simulink model "SimplePendulum"  (R2025b)
settings: Solver=VariableStepAuto  StartTime=0.0  StopTime=10.0  RelTol=1e-3
settings Model: Creator=alvaro  LastModifiedBy=alvaro

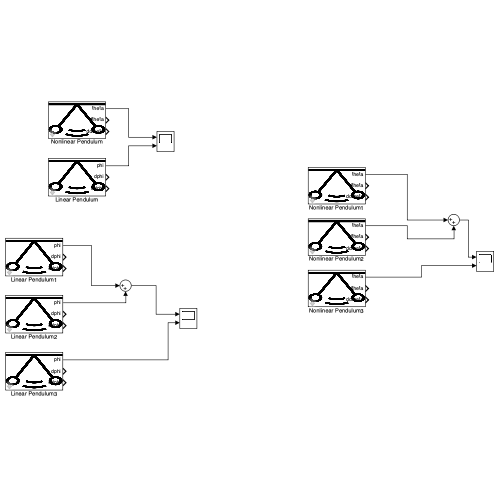
[thumbnail: Simulink's stored preview of the top-level diagram]
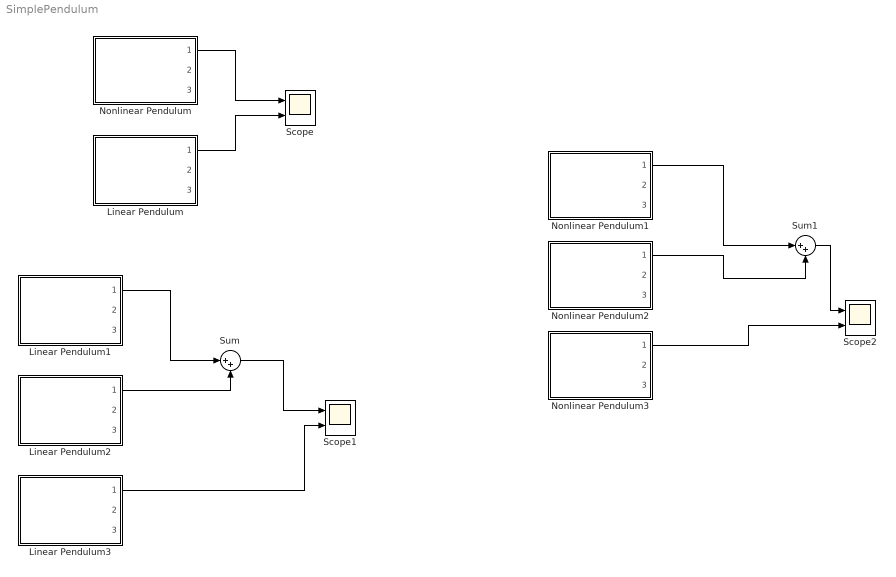
== system SimplePendulum ==
  Linear Pendulum : Subsystem  ReferencedSubsystem=LinearPendulum  b=0.86  g=9.81  l=0.1  phi0=pi/4  dphi0=0
  Linear Pendulum1 : Subsystem  ReferencedSubsystem=LinearPendulum  b=0.86  g=9.81  l=0.1  phi0=0.2  dphi0=0
  Linear Pendulum2 : Subsystem  ReferencedSubsystem=LinearPendulum  b=0.86  g=9.81  l=0.1  phi0=0.2  dphi0=0
  Linear Pendulum3 : Subsystem  ReferencedSubsystem=LinearPendulum  b=0.86  g=9.81  l=0.1  phi0=0.4  dphi0=0
  Nonlinear Pendulum : Subsystem  ReferencedSubsystem=NonlinearPendulum  b=0.86  g=9.81  l=0.1  theta0=pi/4  dtheta0=0
  Nonlinear Pendulum1 : Subsystem  ReferencedSubsystem=NonlinearPendulum  b=0.86  g=9.81  l=0.1  theta0=pi/4  dtheta0=0
  Nonlinear Pendulum2 : Subsystem  ReferencedSubsystem=NonlinearPendulum  b=0.86  g=9.81  l=0.1  theta0=pi/4  dtheta0=0
  Nonlinear Pendulum3 : Subsystem  ReferencedSubsystem=NonlinearPendulum  b=0.86  g=9.81  l=0.1  theta0=pi/2  dtheta0=0
  Scope : Scope  NumInputPorts=2
      settings: ActiveDisplayYMinimum=-1.6985035919332039  ActiveDisplayYMaximum=1.934051873320241
  Scope1 : Scope  NumInputPorts=2
      settings: ActiveDisplayYMinimum=-1.6985035919332039  ActiveDisplayYMaximum=1.934051873320241
  Scope2 : Scope  NumInputPorts=2
      settings: ActiveDisplayYMinimum=-1.6985035919332039  ActiveDisplayYMaximum=1.934051873320241  DataLoggingVariableName=ScopeData2
  Sum : Sum  Inputs=|++
  Sum1 : Sum  Inputs=|++
  wires:
  Nonlinear Pendulum/1 -> Scope/1
  Linear Pendulum/1 -> Scope/2
  Linear Pendulum2/1 -> Sum/2
  Linear Pendulum1/1 -> Sum/1
  Sum/1 -> Scope1/1
  Linear Pendulum3/1 -> Scope1/2
  Nonlinear Pendulum1/1 -> Sum1/1
  Nonlinear Pendulum3/1 -> Scope2/2
  Nonlinear Pendulum2/1 -> Sum1/2
  Sum1/1 -> Scope2/1
